simulink model "TSDa_tClnt"  (R2016b)
settings: configuration reference "CodeGenConfigSet" (kept outside this file)
values from neighbouring files (symbols this model uses):
  TSDa_tRadOutSubs_C = Calibration.Parameter    [init_TSDa_tClnt.m]
settings Model: Creator=xinchangran  LastModifiedBy=xinchangran
settings ConfigSetRef: SourceLocation=Base Workspace

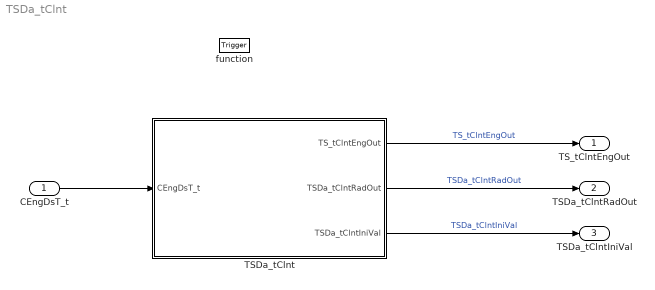
== system TSDa_tClnt ==
  CEngDsT_t : Inport  Tag=deg  Description=engine coolant temperature after filter  OutMin=-200  OutMax=200  OutDataTypeStr=Temp_deg
  function : TriggerPort  TriggerType=function-call  VariantControl=Variant
  TSDa_tClnt : Subsystem
  TS_tClntEngOut : Outport  Tag=deg  Description=Coolant temperature of combustion engine  OutMin=-3549  OutMax=3003  OutDataTypeStr=Temp_deg
  TSDa_tClntRadOut : Outport  Tag=deg  Description=Coolant temperature at radiator outlet  Port=2  OutMin=-3549  OutMax=3003  OutDataTypeStr=Temp_deg
  TSDa_tClntIniVal : Outport  Tag=deg  Description=initial value of coolant temperature at engine outlet  Port=3  OutMin=-3549  OutMax=3003  OutDataTypeStr=Temp_deg
  wires:
  CEngDsT_t/1 -> TSDa_tClnt/1(CEngDsT_t)
  TSDa_tClnt/1(TS_tClntEngOut) -> TS_tClntEngOut/1  "TS_tClntEngOut"
  TSDa_tClnt/2(TSDa_tClntRadOut) -> TSDa_tClntRadOut/1  "TSDa_tClntRadOut"
  TSDa_tClnt/3(TSDa_tClntIniVal) -> TSDa_tClntIniVal/1  "TSDa_tClntIniVal"

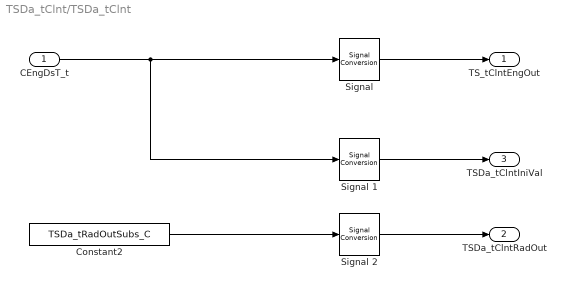
== system TSDa_tClnt/TSDa_tClnt ==
  CEngDsT_t : Inport  Tag=deg  Description=engine coolant temperature after filter  OutMin=-200  OutMax=200  OutDataTypeStr=Temp_deg
  Constant2 : Constant  Value=TSDa_tRadOutSubs_C
  "Signal " : SignalConversion  OverrideOpt=off
  Signal 1 : SignalConversion  OverrideOpt=off
  Signal 2 : SignalConversion  OverrideOpt=off
  TS_tClntEngOut : Outport  Tag=deg  Description=Coolant temperature of combustion engine  OutMin=-3549  OutMax=3003  OutDataTypeStr=Temp_deg
  TSDa_tClntRadOut : Outport  Tag=deg  Description=Coolant temperature at radiator outlet  Port=2  OutMin=-3549  OutMax=3003  OutDataTypeStr=Temp_deg
  TSDa_tClntIniVal : Outport  Tag=deg  Description=initial value of coolant temperature at engine outlet  Port=3  OutMin=-3549  OutMax=3003  OutDataTypeStr=Temp_deg
  wires:
  "Signal "/1 -> TS_tClntEngOut/1
  CEngDsT_t/1 -> Signal 1/1, "Signal "/1
  Constant2/1 -> Signal 2/1
  Signal 1/1 -> TSDa_tClntIniVal/1
  Signal 2/1 -> TSDa_tClntRadOut/1
